simulink model "ImpJoystick"  (R2025b)
settings: Solver=FixedStepAuto  StartTime=0.0  StopTime=inf  FixedStep=Ts  RelTol=1e-3
model workspace (MAT data in the model file):
  SL_ROS_VariableLengthArrays_MaxSizes.CommonInfo.ArrayTruncateAction = 'EmitWarning'
  SL_ROS_VariableLengthArrays_MaxSizes.MsgTypeMap = containers.Map
  SL_ROS_VariableLengthArrays_MaxSizes.MsgTypeMap.serialization.keys = {'sensor_msgs/JointState'}
  SL_ROS_VariableLengthArrays_MaxSizes.MsgTypeMap.serialization.values{1}(1).PropertyName = 'effort'
  SL_ROS_VariableLengthArrays_MaxSizes.MsgTypeMap.serialization.values{1}(1).DataType = 'double'
  SL_ROS_VariableLengthArrays_MaxSizes.MsgTypeMap.serialization.values{1}(1).MaxLength = 3
  SL_ROS_VariableLengthArrays_MaxSizes.MsgTypeMap.serialization.values{1}(2).PropertyName = 'name'
  SL_ROS_VariableLengthArrays_MaxSizes.MsgTypeMap.serialization.values{1}(2).DataType = 'std_msgs/String'
  SL_ROS_VariableLengthArrays_MaxSizes.MsgTypeMap.serialization.values{1}(2).MaxLength = 16
  SL_ROS_VariableLengthArrays_MaxSizes.MsgTypeMap.serialization.values{1}(3).PropertyName = 'position'
  SL_ROS_VariableLengthArrays_MaxSizes.MsgTypeMap.serialization.values{1}(3).DataType = 'double'
  SL_ROS_VariableLengthArrays_MaxSizes.MsgTypeMap.serialization.values{1}(3).MaxLength = 3
  SL_ROS_VariableLengthArrays_MaxSizes.MsgTypeMap.serialization.values{1}(4).PropertyName = 'velocity'
  SL_ROS_VariableLengthArrays_MaxSizes.MsgTypeMap.serialization.values{1}(4).DataType = 'double'
  SL_ROS_VariableLengthArrays_MaxSizes.MsgTypeMap.serialization.values{1}(4).MaxLength = 3
  SL_ROS_VariableLengthArrays_MaxSizes.MsgTypeMap.serialization.uniformity = 0
  SL_ROS_VariableLengthArrays_MaxSizes.MsgTypeMap.serialization.keyType = 'char'
  SL_ROS_VariableLengthArrays_MaxSizes.MsgTypeMap.serialization.valueType = 'any'
values from neighbouring files (symbols this model uses):
  hiddenLayerSizeCtrl = 20    [InitJoystick.m]
  hiddenLayerSizeObsv = 5    [InitJoystick.m]
  p = 3    [InitJoystick.m]
  torque2voltage = voltage_max ./ u_max    [InitJoystick.m]
  Ts = 1e-3    (= 0.001)    [InitJoystick.m]
  u_max = motor_max_torque * gear_ratio    [InitJoystick.m]
  u_min = - motor_max_torque * gear_ratio    [InitJoystick.m]
  Vctrl0 = 0.1 * randn(hiddenLayerSizeCtrl, inputLayerSizeCtrl)    [InitJoystick.m]
  Vobsv0 = 0.1 * randn(hiddenLayerSizeObsv, inputLayerSizeObsv)    [InitJoystick.m]
  Wctrl0 = 0.1 * randn(outputLayerSizeCtrl, hiddenLayerSizeCtrl)    [InitJoystick.m]
  Wobsv0 = 0.1 * randn(outputLayerSizeObsv, hiddenLayerSizeObsv)    [InitJoystick.m]
  x_hat0 = zeros(n, 1)    [InitJoystick.m]
undefined symbols (not defined in the file or in its folder): effort, effort_SL_Info, position, position_SL_Info
libraries: ros2lib x3, slpidlib x3, sl3dlib x1
settings Model: Creator=Asus  LastModifiedBy=Asus
settings OptimizationCC: DefaultParameterBehavior=Inlined  EnhancedBackFolding=on  PassReuseOutputArgsAs=Individual arguments  ZeroExternalMemoryAtStartup=off  ZeroInternalMemoryAtStartup=off  MaxStackSize=64  OptimizeBlockOrder=speed  DifferentSizesBufferReuse=on  OptimizationCustomize=off  EfficientTunableParamExpr=on
settings DebuggingCC: InheritedTsInSrcMsg=none  ParameterTunabilityLossMsg=error
settings SFSimCC: MATLABDynamicMemAlloc=off
settings RTWCC: SystemTargetFile=ert.tlc  HardwareBoard=Robot Operating System 2 (ROS 2)  TLCOptions="-aInlineSetEventsForThisBaseRateFcn=TLC_FALSE -aSuppressMultiTaskScheduler=TLC_FALSE  -aRateBasedStepFcn=0"  TemplateMakefile=ert_default_tmf  Toolchain=Colcon Tools  TargetLang=C++  Description=Embedded Coder
settings CodeAppCC: ForceParamTrailComments=on  IgnoreCustomStorageClasses=off  MaxIdLength=95.0  OperatorAnnotations=on  SimulinkDataObjDesc=on  SFDataObjDesc=on  InsertBlockDesc=on
settings ERTTargetCC: RootIOFormat=Structure reference  CodeInterfacePackaging=C++ class

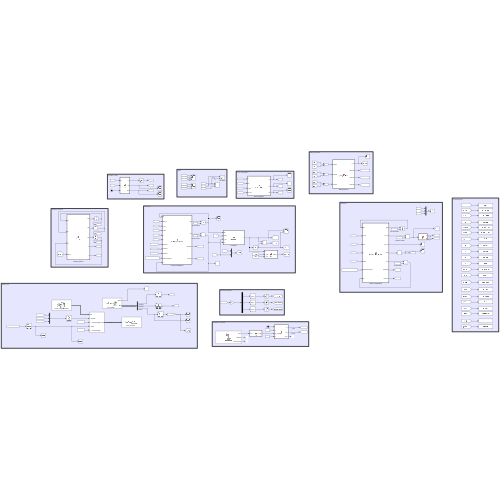
[thumbnail: Simulink's stored preview of the top-level diagram]
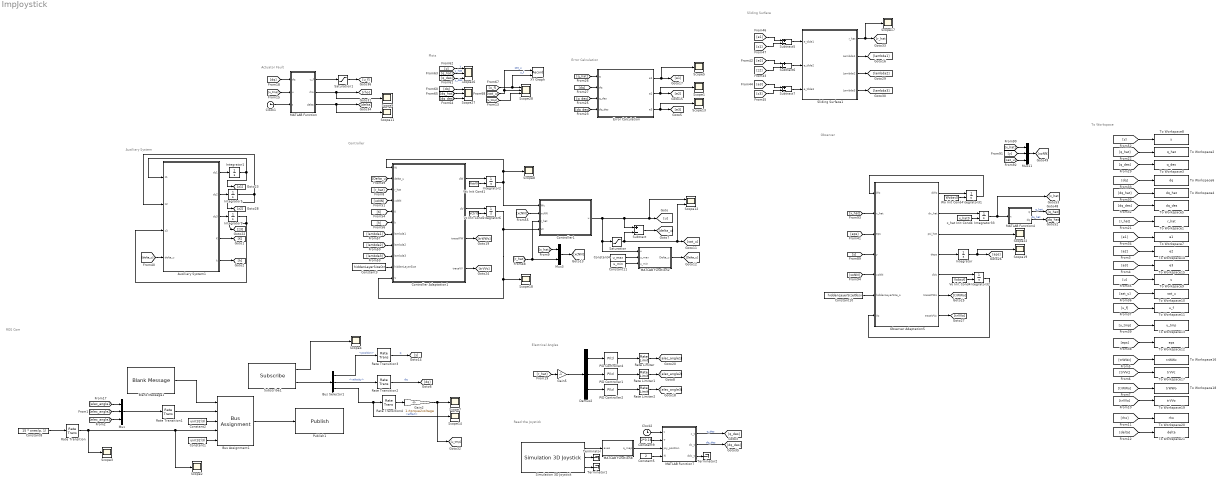
== system ImpJoystick ==
  note: To Workspace
  note: Electrical Angles
  note: Plots
  note: Observer
  note: ROS Com
  note: Actuator Fault
  note: Auxiliary System
  note: Error Calculation
  note: Sliding Surface
  note: Controller
  note: Read the Joystick
  Auxiliary System1 : MATLAB Function  TreatAsAtomicUnit=on
  Blank Message1 : ros2lib/Blank Message  messageClass=Message  entityType=sensor_msgs/JointState  messageType=sensor_msgs/JointState  SampleTime=0.02
  Bus Assignment1 : BusAssignment  AssignedSignals=position,position_SL_Info.CurrentLength,effort,effort_SL_Info.CurrentLength
  Bus Selector1 : BusSelector  OutputSignals=position,velocity,effort
  Clock1 : Clock
  Clock2 : Clock
  Constant1 : Constant  Value=uint32(3)
  Constant10 : Constant  Value=hiddenLayerSizeObsv
  Constant11 : Constant  Value=u_min
  Constant2 : Constant  Value=uint32(3)
  Constant3 : Constant  Value=hiddenLayerSizeCtrl
  Constant4 : Constant  Value=u_max
  Constant5 : Constant  Value=2
  Constant8 : Constant  Value=15 * ones(p, 1)
  Constant9 : Constant  Value=2*0.16
  Controller Adaptation1 : MATLAB Function  TreatAsAtomicUnit=on
  Controller1 : MATLAB Function  TreatAsAtomicUnit=on
  Demux2 : Demux  Outputs=3
  Error Calculation : MATLAB Function  TreatAsAtomicUnit=on
  Gain2 : Gain  Gain=1./torque2voltage
  Gain5 : Gain  Gain=-1
  Integrator : Integrator  InitialCondition=5 * ones(p, 1)
  Integrator1 : Integrator  InitialCondition=zeros(2, 1)
  Integrator{2,6,31..33} (5 alike) : Integrator  InitialConditionSource=external  InitialCondition=[0.5; 0.5]
  Integrator5 : Integrator  InitialCondition=zeros(2, 1)
  Integrator9 : Integrator  InitialCondition=zeros(2, 1)
  MATLAB Function : MATLAB Function  TreatAsAtomicUnit=on
  MATLAB Function2 : MATLAB Function  TreatAsAtomicUnit=on
  MATLAB Function4 : MATLAB Function  TreatAsAtomicUnit=on
  MATLAB Function7 : MATLAB Function  TreatAsAtomicUnit=on  SystemSampleTime=Ts
  MATLAB Function8 : MATLAB Function  TreatAsAtomicUnit=on
  Mux : Mux  Inputs=3
  Mux11 : Mux  Inputs=3
  Mux3 : Mux  Inputs=2
  Observer Adaptation5 : MATLAB Function  TreatAsAtomicUnit=on
  PID Controller1 : slpidlib/PID Controller  Controller=PI  Form=Parallel  TimeDomain=Discrete-time  UseExternalTs=off  SampleTime=-1  IntegratorMethod=Trapezoidal  FilterMethod=Forward Euler  ControllerParametersSource=internal  P=0.05  I=1  UseKiTs=off  D=0  UseExternalDerivativeSource=off  N=100  UseFilter=on  TunerSelectOption=Transfer Function Based (PID Tuner App)  InitialConditionSource=internal  InitialConditionForIntegrator=0  InitialConditionForFilter=0  DifferentiatorICPrevScaledInput=0  ExternalReset=none  TrackingMode=off  Kt=1  LimitOutput=off  SatLimitsSource=internal  UpperSaturationLimit=50  LowerSaturationLimit=-50  LinearizeAsGain=on  AntiWindupMode=none  Kb=1  LimitIntegrator=off  UpperIntegratorSaturationLimit=50  LowerIntegratorSaturationLimit=-50  POutMin=[]  POutMax=[]  IOutMin=[]  IOutMax=[]  DOutMin=[]  DOutMax=[]  NOutMin=[]  NOutMax=[]  SumOutMin=[]  SumOutMax=[]  SaturationOutMin=[]  SaturationOutMax=[]  PParamMin=[]  PParamMax=[]  IParamMin=[]  IParamMax=[]  DParamMin=[]  DParamMax=[]  NParamMin=[]  NParamMax=[]  KbParamMin=[]  KbParamMax=[]  KtParamMin=[]  KtParamMax=[]  KbOutMin=[]  KbOutMax=[]  KtOutMin=[]  KtOutMax=[]  IntegratorOutMin=[]  IntegratorOutMax=[]  FilterOutMin=[]  FilterOutMax=[]  SumI1OutMin=[]  SumI1OutMax=[]  SumI2OutMin=[]  SumI2OutMax=[]  SumI3OutMin=[]  SumI3OutMax=[]  SumI4OutMin=[]  SumI4OutMax=[]  SumDOutMin=[]  SumDOutMax=[]  DifferentiatorOutMin=[]  DifferentiatorOutMax=[]  FilterDiffOutCoefMin=[]  FilterDiffOutCoefMax=[]  ReciprocalOutMin=[]  ReciprocalOutMax=[]  SumDenOutMin=[]  SumDenOutMax=[]  SumNumOutMin=[]  SumNumOutMax=[]  DivideOutMin=[]  DivideOutMax=[]  UdiffTsProdOutMin=[]  UdiffTsProdOutMax=[]  NTsProdOutMin=[]  NTsProdOutMax=[]  UintegralTsProdOutMin=[]  UintegralTsProdOutMax=[]  UngainTsProdOutMin=[]  UngainTsProdOutMax=[]  ClampingZeroOutDataTypeStr=Inherit: Inherit via back propagation  ClampingZeroOutMin=[]  ClampingZeroOutMax=[]  FilterDenConstantOutDataTypeStr=Inherit: Inherit via back propagation  FilterDenConstantOutMin=[]  FilterDenConstantOutMax=[]  PCopyOutDataTypeStr=Inherit: Inherit via back propagation  PCopyOutMin=[]  PCopyOutMax=[]  NCopyOutDataTypeStr=Inherit: Inherit via back propagation  NCopyOutMin=[]  NCopyOutMax=[]  IntegratorContinuousStateAttributes=''  IntegratorStateMustResolveToSignalObject=off  IntegratorRTWStateStorageClass=Auto  FilterContinuousStateAttributes=''  FilterStateMustResolveToSignalObject=off  FilterRTWStateStorageClass=Auto  ParallelPVariant=InternalParameters  IdealPVariant=Disabled  IVariant=InternalParameters  DVariant=Disabled  IntegratorVariant=Discrete  SatVariant=Disabled  AWVariant=Passthrough  PCopyVariant=Disabled  TRVariant=Disabled  FdbkBlocksVariant=Forward  IdealPFdbkVariant=Disabled  SatFdbkVariant=Disabled  DerivativeFilterVariant=Disabled  NVariant=Disabled  NCopyVariant=Disabled_SignalSpec  FilterICVariant=Disabled  IntegratorICVariant=InternalICs  ExternalResetVariant=Disabled  TRSumVariant=Passthrough  SumFdbkVariant=Disabled  SumVariant=Sum_PI  TsampFilterVariant=InternalTs  TsampNgainVariant=Passthrough  TsampIntegralVariant=Disabled_SignalSpec  ExternalSaturationOutDataTypeStr=Inherit: Same as second input  DerivativeSourceVariant=Disabled  PreIntVariant=InternalPreInt
  PID Controller2 : slpidlib/PID Controller  Controller=PI  Form=Parallel  TimeDomain=Discrete-time  UseExternalTs=off  SampleTime=-1  IntegratorMethod=Trapezoidal  FilterMethod=Forward Euler  ControllerParametersSource=internal  P=0.05  I=1  UseKiTs=off  D=0  UseExternalDerivativeSource=off  N=100  UseFilter=on  TunerSelectOption=Transfer Function Based (PID Tuner App)  InitialConditionSource=internal  InitialConditionForIntegrator=0  InitialConditionForFilter=0  DifferentiatorICPrevScaledInput=0  ExternalReset=none  TrackingMode=off  Kt=1  LimitOutput=off  SatLimitsSource=internal  UpperSaturationLimit=50  LowerSaturationLimit=-50  LinearizeAsGain=on  AntiWindupMode=none  Kb=1  LimitIntegrator=off  UpperIntegratorSaturationLimit=50  LowerIntegratorSaturationLimit=-50  POutMin=[]  POutMax=[]  IOutMin=[]  IOutMax=[]  DOutMin=[]  DOutMax=[]  NOutMin=[]  NOutMax=[]  SumOutMin=[]  SumOutMax=[]  SaturationOutMin=[]  SaturationOutMax=[]  PParamMin=[]  PParamMax=[]  IParamMin=[]  IParamMax=[]  DParamMin=[]  DParamMax=[]  NParamMin=[]  NParamMax=[]  KbParamMin=[]  KbParamMax=[]  KtParamMin=[]  KtParamMax=[]  KbOutMin=[]  KbOutMax=[]  KtOutMin=[]  KtOutMax=[]  IntegratorOutMin=[]  IntegratorOutMax=[]  FilterOutMin=[]  FilterOutMax=[]  SumI1OutMin=[]  SumI1OutMax=[]  SumI2OutMin=[]  SumI2OutMax=[]  SumI3OutMin=[]  SumI3OutMax=[]  SumI4OutMin=[]  SumI4OutMax=[]  SumDOutMin=[]  SumDOutMax=[]  DifferentiatorOutMin=[]  DifferentiatorOutMax=[]  FilterDiffOutCoefMin=[]  FilterDiffOutCoefMax=[]  ReciprocalOutMin=[]  ReciprocalOutMax=[]  SumDenOutMin=[]  SumDenOutMax=[]  SumNumOutMin=[]  SumNumOutMax=[]  DivideOutMin=[]  DivideOutMax=[]  UdiffTsProdOutMin=[]  UdiffTsProdOutMax=[]  NTsProdOutMin=[]  NTsProdOutMax=[]  UintegralTsProdOutMin=[]  UintegralTsProdOutMax=[]  UngainTsProdOutMin=[]  UngainTsProdOutMax=[]  ClampingZeroOutDataTypeStr=Inherit: Inherit via back propagation  ClampingZeroOutMin=[]  ClampingZeroOutMax=[]  FilterDenConstantOutDataTypeStr=Inherit: Inherit via back propagation  FilterDenConstantOutMin=[]  FilterDenConstantOutMax=[]  PCopyOutDataTypeStr=Inherit: Inherit via back propagation  PCopyOutMin=[]  PCopyOutMax=[]  NCopyOutDataTypeStr=Inherit: Inherit via back propagation  NCopyOutMin=[]  NCopyOutMax=[]  IntegratorContinuousStateAttributes=''  IntegratorStateMustResolveToSignalObject=off  IntegratorRTWStateStorageClass=Auto  FilterContinuousStateAttributes=''  FilterStateMustResolveToSignalObject=off  FilterRTWStateStorageClass=Auto  ParallelPVariant=InternalParameters  IdealPVariant=Disabled  IVariant=InternalParameters  DVariant=Disabled  IntegratorVariant=Discrete  SatVariant=Disabled  AWVariant=Passthrough  PCopyVariant=Disabled  TRVariant=Disabled  FdbkBlocksVariant=Forward  IdealPFdbkVariant=Disabled  SatFdbkVariant=Disabled  DerivativeFilterVariant=Disabled  NVariant=Disabled  NCopyVariant=Disabled_SignalSpec  FilterICVariant=Disabled  IntegratorICVariant=InternalICs  ExternalResetVariant=Disabled  TRSumVariant=Passthrough  SumFdbkVariant=Disabled  SumVariant=Sum_PI  TsampFilterVariant=InternalTs  TsampNgainVariant=Passthrough  TsampIntegralVariant=Disabled_SignalSpec  ExternalSaturationOutDataTypeStr=Inherit: Same as second input  DerivativeSourceVariant=Disabled  PreIntVariant=InternalPreInt
  PID Controller4 : slpidlib/PID Controller  Controller=PI  Form=Parallel  TimeDomain=Discrete-time  UseExternalTs=off  SampleTime=-1  IntegratorMethod=Trapezoidal  FilterMethod=Forward Euler  ControllerParametersSource=internal  P=0.05  I=1  UseKiTs=off  D=0  UseExternalDerivativeSource=off  N=100  UseFilter=on  TunerSelectOption=Transfer Function Based (PID Tuner App)  InitialConditionSource=internal  InitialConditionForIntegrator=0  InitialConditionForFilter=0  DifferentiatorICPrevScaledInput=0  ExternalReset=none  TrackingMode=off  Kt=1  LimitOutput=off  SatLimitsSource=internal  UpperSaturationLimit=50  LowerSaturationLimit=-50  LinearizeAsGain=on  AntiWindupMode=none  Kb=1  LimitIntegrator=off  UpperIntegratorSaturationLimit=50  LowerIntegratorSaturationLimit=-50  POutMin=[]  POutMax=[]  IOutMin=[]  IOutMax=[]  DOutMin=[]  DOutMax=[]  NOutMin=[]  NOutMax=[]  SumOutMin=[]  SumOutMax=[]  SaturationOutMin=[]  SaturationOutMax=[]  PParamMin=[]  PParamMax=[]  IParamMin=[]  IParamMax=[]  DParamMin=[]  DParamMax=[]  NParamMin=[]  NParamMax=[]  KbParamMin=[]  KbParamMax=[]  KtParamMin=[]  KtParamMax=[]  KbOutMin=[]  KbOutMax=[]  KtOutMin=[]  KtOutMax=[]  IntegratorOutMin=[]  IntegratorOutMax=[]  FilterOutMin=[]  FilterOutMax=[]  SumI1OutMin=[]  SumI1OutMax=[]  SumI2OutMin=[]  SumI2OutMax=[]  SumI3OutMin=[]  SumI3OutMax=[]  SumI4OutMin=[]  SumI4OutMax=[]  SumDOutMin=[]  SumDOutMax=[]  DifferentiatorOutMin=[]  DifferentiatorOutMax=[]  FilterDiffOutCoefMin=[]  FilterDiffOutCoefMax=[]  ReciprocalOutMin=[]  ReciprocalOutMax=[]  SumDenOutMin=[]  SumDenOutMax=[]  SumNumOutMin=[]  SumNumOutMax=[]  DivideOutMin=[]  DivideOutMax=[]  UdiffTsProdOutMin=[]  UdiffTsProdOutMax=[]  NTsProdOutMin=[]  NTsProdOutMax=[]  UintegralTsProdOutMin=[]  UintegralTsProdOutMax=[]  UngainTsProdOutMin=[]  UngainTsProdOutMax=[]  ClampingZeroOutDataTypeStr=Inherit: Inherit via back propagation  ClampingZeroOutMin=[]  ClampingZeroOutMax=[]  FilterDenConstantOutDataTypeStr=Inherit: Inherit via back propagation  FilterDenConstantOutMin=[]  FilterDenConstantOutMax=[]  PCopyOutDataTypeStr=Inherit: Inherit via back propagation  PCopyOutMin=[]  PCopyOutMax=[]  NCopyOutDataTypeStr=Inherit: Inherit via back propagation  NCopyOutMin=[]  NCopyOutMax=[]  IntegratorContinuousStateAttributes=''  IntegratorStateMustResolveToSignalObject=off  IntegratorRTWStateStorageClass=Auto  FilterContinuousStateAttributes=''  FilterStateMustResolveToSignalObject=off  FilterRTWStateStorageClass=Auto  ParallelPVariant=InternalParameters  IdealPVariant=Disabled  IVariant=InternalParameters  DVariant=Disabled  IntegratorVariant=Discrete  SatVariant=Disabled  AWVariant=Passthrough  PCopyVariant=Disabled  TRVariant=Disabled  FdbkBlocksVariant=Forward  IdealPFdbkVariant=Disabled  SatFdbkVariant=Disabled  DerivativeFilterVariant=Disabled  NVariant=Disabled  NCopyVariant=Disabled_SignalSpec  FilterICVariant=Disabled  IntegratorICVariant=InternalICs  ExternalResetVariant=Disabled  TRSumVariant=Passthrough  SumFdbkVariant=Disabled  SumVariant=Sum_PI  TsampFilterVariant=InternalTs  TsampNgainVariant=Passthrough  TsampIntegralVariant=Disabled_SignalSpec  ExternalSaturationOutDataTypeStr=Inherit: Same as second input  DerivativeSourceVariant=Disabled  PreIntVariant=InternalPreInt
  Publish1 : ros2lib/Publish  topicSource=Specify your own  topic=/joint_desireds  messageType=sensor_msgs/JointState  QOSHistory=Keep last  QOSDepth=10  QOSReliability=Reliable  QOSDurability=Volatile  QOSDeadline=Inf  QOSLifespan=Inf  QOSLiveliness=Automatic  QOSLeaseDuration=Inf  QOSAvoidROSNamespaceConventions=off
  Rate Limiter : RateLimiter  RisingSlewLimit=50  FallingSlewLimit=-50
  Rate Limiter1 : RateLimiter  RisingSlewLimit=50  FallingSlewLimit=-50  SampleTimeMode=inherited
  Rate Limiter2 : RateLimiter  RisingSlewLimit=50  FallingSlewLimit=-50  SampleTimeMode=inherited
  Rate Transition : RateTransition  OutPortSampleTime=0.02
  Rate Transition1 : RateTransition  OutPortSampleTime=0.02
  Rate Transition2 : RateTransition  OutPortSampleTime=Ts
  Rate Transition3 : RateTransition  OutPortSampleTime=Ts
  Rate Transition4 : RateTransition  OutPortSampleTime=Ts
  Saturation : Saturate  UpperLimit=u_max  LowerLimit=u_min
  Saturation1 : Saturate  UpperLimit=u_max  LowerLimit=u_min
  Scope{1..5,7..9,11,13..14,17..19,22} (15 alike) : Scope
      Scope1 settings: ActiveDisplayYMinimum=-0.24287807344006263  ActiveDisplayYMaximum=0.25287974310957717  DataLoggingVariableName=ScopeData3
      Scope11 settings: ActiveDisplayYMinimum=-1  ActiveDisplayYMaximum=1  DataLoggingVariableName=ScopeData6
      Scope13 settings: ActiveDisplayYMinimum=-0.29897924911149121  ActiveDisplayYMaximum=0.2090765790905024  DataLoggingVariableName=ScopeData13
      Scope14 settings: ActiveDisplayYMinimum=-12.649985074996948  ActiveDisplayYMaximum=12.652279615402222  DataLoggingVariableName=ScopeData14
      Scope17 settings: ActiveDisplayYMinimum=-6.84986892680592  ActiveDisplayYMaximum=3.4555315948976819  DataLoggingVariableName=ScopeData19
      Scope18 settings: ActiveDisplayYMinimum=-1  ActiveDisplayYMaximum=1  DataLoggingVariableName=ScopeData10
      Scope19 settings: ActiveDisplayYMinimum=-0.056716812017258533  ActiveDisplayYMaximum=20.510451308155332  DataLoggingVariableName=ScopeData15
      Scope2 settings: ActiveDisplayYMinimum=-1.8749999999999996  ActiveDisplayYMaximum=16.875
      Scope22 settings: ActiveDisplayYMinimum=-0.42606678523590263  ActiveDisplayYMaximum=0.48150686097965856  DataLoggingVariableName=ScopeData18
      Scope3 settings: ActiveDisplayYMinimum=5  ActiveDisplayYMaximum=25  DataLoggingVariableName=ScopeData4
      Scope4 settings: ActiveDisplayYMinimum=-0.12499999999999997  ActiveDisplayYMaximum=1.125  DataLoggingVariableName=ScopeData11
      Scope5 settings: ActiveDisplayYMinimum=-5.0160610234879295  ActiveDisplayYMaximum=4.3832959736672761
      Scope7 settings: ActiveDisplayYMinimum=-4.6454817136128748  ActiveDisplayYMaximum=4.6375481605529787  DataLoggingVariableName=ScopeData8
      Scope8 settings: ActiveDisplayYMinimum=-68.998192796896234  ActiveDisplayYMaximum=67.9276309158068  DataLoggingVariableName=ScopeData20
      Scope9 settings: ActiveDisplayYMinimum=0.89735957983734793  ActiveDisplayYMaximum=1.3932448974534157  DataLoggingVariableName=ScopeData5
  Scope12 : Scope  NumInputPorts=2
      settings: ActiveDisplayYMinimum=-6.9909348188181673  ActiveDisplayYMaximum=6.9347067315860729  DataLoggingVariableName=ScopeData7
  Scope26 : Scope  NumInputPorts=3
      settings: ActiveDisplayYMinimum=-0.16267971265796272  ActiveDisplayYMaximum=0.24936946493277015  DataLoggingVariableName=ScopeData22
  Scope27 : Scope  NumInputPorts=3
      settings: ActiveDisplayYMinimum=-0.15237484375  ActiveDisplayYMaximum=0.27574859375000021  DataLoggingVariableName=ScopeData23
  Scope28 : Scope  NumInputPorts=3
      settings: ActiveDisplayYMinimum=-1.7792114485048884  ActiveDisplayYMaximum=0.75655926497715087  DataLoggingVariableName=ScopeData24
  Simulation 3D Joystick : sl3dlib/Simulation 3D/Hardware Interface/Simulation 3D Joystick  joyid=1  adjustports=on  forcefeed=off
  Sliding Surface1 : MATLAB Function  TreatAsAtomicUnit=on
  Subscribe1 : ros2lib/Subscribe  topicSource=Select from ROS network  topic=/joint_states  messageType=sensor_msgs/JointState  sampleTime=0.02  QOSHistory=Keep all  QOSDepth=3  QOSReliability=Best effort  QOSDurability=Volatile  QOSDeadline=Inf  QOSLifespan=Inf  QOSLiveliness=Automatic  QOSLeaseDuration=Inf  QOSAvoidROSNamespaceConventions=off
  Subtract{,5..7} (4 alike) : Sum  Inputs=+-
  Terminator : Terminator
  Terminator1 : Terminator
  Terminator2 : Terminator
  To Workspace1 : ToWorkspace  VariableName=r_hat  SaveFormat=Structure  SampleTime=-1
      settings: Save2DSignal=2-D array (concatenate along first dimension)
  To Workspace10 : ToWorkspace  VariableName=sat_u  SaveFormat=Structure  SampleTime=-1
      settings: Save2DSignal=2-D array (concatenate along first dimension)
  To Workspace11 : ToWorkspace  VariableName=u_f  SaveFormat=Structure  SampleTime=-1
      settings: Save2DSignal=2-D array (concatenate along first dimension)
  To Workspace12 : ToWorkspace  VariableName=eps  SaveFormat=Structure  SampleTime=-1
      settings: Save2DSignal=2-D array (concatenate along first dimension)
  To Workspace13 : ToWorkspace  VariableName=u_tmp  SaveFormat=Structure  SampleTime=-1
      settings: Save2DSignal=2-D array (concatenate along first dimension)
  To Workspace14 : ToWorkspace  VariableName=e2  SaveFormat=Structure  SampleTime=-1
      settings: Save2DSignal=2-D array (concatenate along first dimension)
  To Workspace15 : ToWorkspace  VariableName=e3  SaveFormat=Structure  SampleTime=-1
      settings: Save2DSignal=2-D array (concatenate along first dimension)
  To Workspace16 : ToWorkspace  VariableName=trWWc  SaveFormat=Structure  SampleTime=-1
      settings: Save2DSignal=2-D array (concatenate along first dimension)
  To Workspace17 : ToWorkspace  VariableName=trVVc  SaveFormat=Structure  SampleTime=-1
      settings: Save2DSignal=2-D array (concatenate along first dimension)
  To Workspace18 : ToWorkspace  VariableName=trWWo  SaveFormat=Structure  SampleTime=-1
      settings: Save2DSignal=2-D array (concatenate along first dimension)
  To Workspace19 : ToWorkspace  VariableName=trVVo  SaveFormat=Structure  SampleTime=-1
      settings: Save2DSignal=2-D array (concatenate along first dimension)
  To Workspace2 : ToWorkspace  VariableName=q_hat  SaveFormat=Structure  SampleTime=-1
      settings: Save2DSignal=2-D array (concatenate along first dimension)
  To Workspace20 : ToWorkspace  VariableName=rho  SaveFormat=Structure  SampleTime=-1
      settings: Save2DSignal=2-D array (concatenate along first dimension)
  To Workspace21 : ToWorkspace  VariableName=delta  SaveFormat=Structure  SampleTime=-1
      settings: Save2DSignal=2-D array (concatenate along first dimension)
  To Workspace3 : ToWorkspace  VariableName=q_des  SaveFormat=Structure  SampleTime=-1
      settings: Save2DSignal=2-D array (concatenate along first dimension)
  To Workspace4 : ToWorkspace  VariableName=dq_hat  SaveFormat=Structure  SampleTime=-1
      settings: Save2DSignal=2-D array (concatenate along first dimension)
  To Workspace5 : ToWorkspace  VariableName=dq_des  SaveFormat=Structure  SampleTime=-1
      settings: Save2DSignal=2-D array (concatenate along first dimension)
  To Workspace6 : ToWorkspace  VariableName=dq  SaveFormat=Structure  SampleTime=-1
      settings: Save2DSignal=2-D array (concatenate along first dimension)
  To Workspace7 : ToWorkspace  VariableName=e1  SaveFormat=Structure  SampleTime=-1
      settings: Save2DSignal=2-D array (concatenate along first dimension)
  To Workspace8 : ToWorkspace  VariableName=y  SaveFormat=Structure  SampleTime=-1
      settings: Save2DSignal=2-D array (concatenate along first dimension)
  To Workspace9 : ToWorkspace  VariableName=u  SaveFormat=Structure  SampleTime=-1
      settings: Save2DSignal=2-D array (concatenate along first dimension)
  Vc Init Cond1 : Constant  Value=Vctrl0
  Vo Init Cond4 : Constant  Value=Vobsv0
  Wc Init Cond1 : Constant  Value=Wctrl0
  Wo Init Cond4 : Constant  Value=Wobsv0
  XY Graph : Record  NumPorts=2.0  FileSettingsInternal="{\"entries\":[{\"content\":{\"excelSettings\":{\"content\":{},\"type\":\"Streamout.ExcelSettings\"},\"parquetSettings\":{\"content\":{},\"type\":\"Streamout.ParquetSettings\"}},\"type\":\"Streamout.FileSettingStorage\",\"uuid\":\"\"}],\"packageUris\":[\"http:\\/\\/schema.mathworks.com\\/mf0\\/streamout_blocks\\/R2020a\"],\"version\":\"1.0\"}"  FrameSettings=[0, 0]  Layout=[1 1]  SignalsInternal="{\"entries\":[{\"content\":{\"signals\":[{\"content\":{\"blockPath\":[],\"dimensions\":[3,1],\"domain\":\"\",\"hasChildren\":true,\"lineColor\":\"#ff6929\",\"lineWidth\":2,\"port\":1,\"signalID\":1,\"signalName\":\"sat_u\"},\"type\":\"RecordBlkView.Signal\",\"uuid\":\"\"},{\"content\":{\"blockPath\":[],\"channel\":[1,1],\"dimensions\":[3,1],\"domain\":\"\",\"lineColor\":\"#64d413\",\"lineWidth\":2,\"parentID\":1,\"port\":1,\"signalID\":2,\"signalName\":\"sat_u\"},\"type\":\"RecordBlkView.Signal\",\"uuid\":\"\"},{\"content\":{\"blockPath\":[],\"channel\":[2,1],\"dimensions\":[3,1],\"domain\":\"\",\"lineColor\":\"#d95319\",\"lineWidth\":2,\"parentID\":1,\"plots\":[ 1 ],\"port\":1,\"signalID\":3,\"signalName\":\"sat_u\"},\"type\":\"RecordBlkView.Signal\",\"uuid\":\"\"},{\"content\":{\"blockPath\":[],\"channel\":[3,1],\"dimensions\":[3,1],\"domain\":\"\",\"lineColor\":\"#edb120\",\"lineWidth\":2,\"parentID\":1,\"port\":1,\"signalID\":4,\"signalName\":\"sat_u\"},\"type\":\"RecordBlkView.Signal\",\"uuid\":\"\"},{\"content\":{\"blockPath\":[],\"dimensions\":[3,1],\"domain\":\"\",\"hasChildren\":true,\"lineColor\":\"#64d413\",\"lineWidth\":2,\"port\":2,\"signalID\":5,\"signalName\":\"u_f\"},\"type\":\"RecordBlkView.Signal\",\"uuid\":\"\"},{\"content\":{\"blockPath\":[],\"channel\":[1,1],\"dimensions\":[3,1],\"domain\":\"\",\"lineColor\":\"#fe330a\",\"lineWidth\":2,\"parentID\":5,\"port\":2,\"signalID\":6,\"signalName\":\"u_f\"},\"type\":\"RecordBlkView.Signal\",\"uuid\":\"\"},{\"content\":{\"blockPath\":[],\"channel\":[2,1],\"dimensions\":[3,1],\"domain\":\"\",\"lineColor\":\"#7e2f8e\",\"lineWidth\":2,\"parentID\":5,\"plots\":[ 1 ],\"port\":2,\"signalID\":7,\"signalName\":\"u_f\"},\"type\":\"RecordBlkView.Signal\",\"uuid\":\"\"},{\"content\":{\"blockPath\":[],\"channel\":[3,1],\"dimensions\":[3,1],\"domain\":\"\",\"lineColor\":\"#77ac30\",\"lineWidth\":2,\"parentID\":5,\"port\":2,\"signalID\":8,\"signalName\":\"u_f\"},\"type\":\"RecordBlkView.Signal\",\"uuid\":\"\"}]},\"type\":\"RecordBlkView.InputSignals\",\"uuid\":\"\"}],\"packageUris\":[\"http:\\/\\/schema.mathworks.com\\/mf0\\/streamout_blocks\\/R2020a\"],\"version\":\"1.0\"}"  VisualizationBindings="{\"xyplotplugin\":{\"info\":[{\"series\":[{\"bindingParametersList\":[{\"parameter\":\"X-Axis\",\"signalID\":3,\"signalName\":\"sat_u(2,1)\"},{\"parameter\":\"Y-Axis\",\"signalID\":7,\"signalName\":\"u_f(2,1)\"}],\"seriesID\":0}],\"subplotID\":1}]}}"  CompatibilityTag=XY
  x_hat Init Cond4 : Constant  Value=x_hat0
  wires:
  Mux/1 -> Rate Transition1/1
  Blank Message1/1 -> Bus Assignment1/1
  Integrator31/1 -> Observer Adaptation5/1(Wo)
  Wo Init Cond4/1 -> Integrator31/2
  Bus Selector1/2 -> Rate Transition2/1  "<velocity>"
  Observer Adaptation5/4(deps) -> Integrator/1
  Vo Init Cond4/1 -> Integrator32/2
  [x_hat] -> Observer Adaptation5/2(x_hat)
  [dq] -> MATLAB Function/1(dq)
  Bus Assignment1/1 -> Publish1/1
  MATLAB Function/2(rho) -> [rho], Scope9/1
  [y] -> Observer Adaptation5/4(y)
  MATLAB Function/3(delta) -> [delta], Scope11/1
  [eps] -> Observer Adaptation5/3(eps)
  [sat_u] -> Mux11/3
  Clock1/1 -> MATLAB Function/3(t)
  [dq_des] -> Scope27/3
  MATLAB Function4/1(q) -> [q_hat]  "q_hat"
  [u_tmp] -> MATLAB Function/2(u)
  Bus Selector1/1 -> Rate Transition3/1  "<position>"
  [q_des] -> Scope26/3  "y_des"
  Rate Transition1/1 -> Bus Assignment1/2
  Observer Adaptation5/1(dWo) -> Integrator31/1
  Constant1/1 -> Bus Assignment1/5
  MATLAB Function/1(u_f) -> Saturation1/1
  Constant10/1 -> Observer Adaptation5/6(hiddenLayerSize_o)
  [x_hat] -> Mux11/1
  [y] -> Mux11/2
  Integrator/1 -> Scope19/1, [eps]
  Observer Adaptation5/2(dx_hat) -> Integrator33/1
  Integrator32/1 -> Observer Adaptation5/7(Vo)
  MATLAB Function4/2(dq) -> [dq_hat]  "dq_hat"
  Subscribe1/1 -> Scope4/1
  [dq] -> Scope27/1
  [q_hat] -> Scope26/2  "y_hat"
  [u_f] -> XY Graph/2, Scope28/1  "u_f"
  [dq_hat] -> Scope27/2
  Subscribe1/2 -> Bus Selector1/1
  [xoNN] -> Observer Adaptation5/5(xoNN)
  x_hat Init Cond4/1 -> Integrator33/2
  [y] -> Scope26/1  "y"
  Observer Adaptation5/3(psi_hat) -> Scope22/1
  Saturation1/1 -> [u_f]
  [sat_u] -> XY Graph/1, Scope28/2  "sat_u"
  Mux11/1 -> [xoNN]
  Rate Transition4/1 -> Gain2/1
  Observer Adaptation5/5(dVo) -> Integrator32/1
  Bus Selector1/3 -> Scope14/1, Rate Transition4/1  "<effort>"
  Constant2/1 -> Bus Assignment1/3
  Integrator33/1 -> MATLAB Function4/1(x), [x_hat]
  Gain2/1 -> [u_tmp], Scope7/1
  Rate Transition/1 -> Scope2/1, Bus Assignment1/4, Scope3/1
  Rate Limiter/1 -> [elec_angle1]
  PID Controller4/1 -> Rate Limiter/1
  [y] -> To Workspace8/1
  [r_hat] -> To Workspace1/1
  [q_hat] -> To Workspace2/1
  [q_des] -> To Workspace3/1
  [dq_hat] -> To Workspace4/1
  [dq] -> To Workspace6/1
  [dq_des] -> To Workspace5/1
  [e1] -> To Workspace7/1
  [u] -> To Workspace9/1
  [sat_u] -> To Workspace10/1
  [u_f] -> To Workspace11/1
  [eps] -> To Workspace12/1
  [u_tmp] -> To Workspace13/1
  Auxiliary System1/1(dz1) -> Integrator1/1
  Auxiliary System1/3(dz3) -> Integrator9/1
  Auxiliary System1/2(dz2) -> Integrator5/1
  Integrator5/1 -> [z2], Auxiliary System1/2(z2)
  Auxiliary System1/5(h) -> [h]
  Integrator9/1 -> Auxiliary System1/3(z3), [z3]
  [delta_u] -> Auxiliary System1/4(delta_u)
  Integrator1/1 -> [z1], Auxiliary System1/1(z1)
  Auxiliary System1/4(K) -> [K]
  Error Calculation/2(e2) -> [e2], Scope1/1
  Error Calculation/1(e1) -> [e1], Scope5/1
  Error Calculation/3(e3) -> Scope13/1, [e3]
  [dq] -> Error Calculation/2(dq)
  [dq_des] -> Error Calculation/4(dq_des)
  [q_hat] -> Error Calculation/1(q)
  [q_des] -> Error Calculation/3(q_des)
  [z1] -> Subtract5/2
  Subtract6/1 -> Sliding Surface1/2(e_tilde2)
  [z3] -> Subtract7/2
  Sliding Surface1/3(Lambda2) -> [lambda2]
  Sliding Surface1/4(Lambda3) -> [lambda3]
  Sliding Surface1/2(Lambda1) -> [lambda1]
  Subtract7/1 -> Sliding Surface1/3(e_tilde3)
  Subtract5/1 -> Sliding Surface1/1(e_tilde1)
  Sliding Surface1/1(r_hat) -> Scope17/1, [r_hat]
  [e3] -> Subtract7/1
  [e1] -> Subtract5/1
  [e2] -> Subtract6/1
  [z2] -> Subtract6/2
  [r_hat] -> Controller Adaptation1/3(r_hat)
  Controller Adaptation1/2(dV) -> Integrator6/1
  MATLAB Function2/1(Delta_u) -> [Delta_u]
  Integrator2/1 -> Controller1/1(Wc), Scope8/1, Controller Adaptation1/1(W)
  [lambda3] -> Controller Adaptation1/9(lambda3)
  [xcNN] -> Controller Adaptation1/4(xcNN)
  Controller Adaptation1/1(dW) -> Integrator2/1
  Constant4/1 -> MATLAB Function2/2(u_max)
  [lambda2] -> Controller Adaptation1/8(lambda2)
  [r_hat] -> Controller1/3(r_hat), Mux3/2
  [Delta_u] -> Controller Adaptation1/2(delta_u)
  Constant11/1 -> MATLAB Function2/3(u_min)
  [lambda1] -> Controller Adaptation1/7(lambda1)
  Wc Init Cond1/1 -> Integrator2/2
  Subtract/1 -> [delta_u]
  [h] -> Controller Adaptation1/6(h)
  Vc Init Cond1/1 -> Integrator6/2
  Mux3/1 -> [xcNN]
  [xcNN] -> Controller1/2(xcNN)
  Controller1/1(u) -> Scope12/1, [u], Subtract/1, MATLAB Function2/1(u), Saturation/1
  [x_hat] -> Mux3/1
  [K] -> Controller Adaptation1/5(K)
  Constant3/1 -> Controller Adaptation1/10(hiddenLayerSize)
  Integrator6/1 -> Scope18/1, Controller Adaptation1/11(V), Controller1/4(Vc)
  Saturation/1 -> Scope12/2, [sat_u], Subtract/2
  PID Controller1/1 -> Rate Limiter1/1
  Rate Limiter1/1 -> [elec_angle2]
  PID Controller2/1 -> Rate Limiter2/1
  Rate Limiter2/1 -> [elec_angle3]
  [elec_angle3] -> Mux/3
  [elec_angle2] -> Mux/2
  [e2] -> To Workspace14/1
  [e3] -> To Workspace15/1
  Rate Transition3/1 -> [y]  "q"
  Rate Transition2/1 -> [dq]  "dq"
  Controller Adaptation1/3(traceWW) -> [trWWc]
  Controller Adaptation1/4(traceVV) -> [trVVc]
  Observer Adaptation5/6(traceWWo) -> [trWWo]
  Observer Adaptation5/7(traceVVo) -> [trVVo]
  [trWWc] -> To Workspace16/1
  [trVVc] -> To Workspace17/1
  [trVVo] -> To Workspace19/1
  [trWWo] -> To Workspace18/1
  [rho] -> To Workspace20/1
  [delta] -> To Workspace21/1
  [elec_angle1] -> Mux/1
  Constant8/1 -> Rate Transition/1
  Demux2/1 -> PID Controller4/1
  Demux2/2 -> PID Controller1/1
  Demux2/3 -> PID Controller2/1
  Simulation 3D Joystick/1 -> MATLAB Function8/1(axes)
  Constant9/1 -> MATLAB Function7/2(T)
  MATLAB Function7/3(ddx_t) -> Terminator2/1
  Simulation 3D Joystick/3 -> Terminator1/1
  Simulation 3D Joystick/2 -> Terminator/1
  MATLAB Function8/1(q_map) -> MATLAB Function7/3(joy_position)
  Clock2/1 -> MATLAB Function7/1(t)
  [u_tmp] -> Scope28/3
  MATLAB Function7/1(x_t) -> [q_des]  "q_des"
  Constant5/1 -> MATLAB Function7/4(N)
  MATLAB Function7/2(dx_t) -> [dq_des]  "dq_des"
  [r_hat] -> Gain5/1
  Gain5/1 -> Demux2/1

== matlab function ImpJoystick/Controller Adaptation1 ==
  data: dW output; dV output; W input; delta_u input; r_hat input; xcNN input; K input; h input; lambda1 input; lambda2 input; lambda3 input; hiddenLayerSize input; V input; traceWW output; traceVV output
function [dW, dV, traceWW, traceVV] = ControllerAdaptation(W, delta_u, r_hat, xcNN, K, h, lambda1, lambda2, lambda3, hiddenLayerSize, V)
    
    Sigma = @(z) (-1 + 2 ./ (1 + exp(-2 * z)));


    l = 20 * [2; 2; 2];

    A1 = [0, 1; 0, 0];
    A2 = [0, 1; 0, 0];
    A3 = [0, 1; 0, 0];

    B1 = [0; 1];
    B2 = [0; 1];
    B3 = [0; 1];

    Ac1 = A1 - B1 * ([lambda1', 1] * l(1) + [0, lambda1']);
    Ac2 = A2 - B2 * ([lambda2', 1] * l(2) + [0, lambda2']);
    Ac3 = A3 - B3 * ([lambda3', 1] * l(3) + [0, lambda3']);

    Ac = blkdiag(Ac1, Ac2, Ac3);
    B  = blkdiag(B1, B2, B3);

    eta   = 10 * [0.1, 0.1];
    gamma = [0.0001, 0.0001];

    PI_c      = diag(Sigma(V * xcNN).^2);
    PI_lambda = blkdiag([lambda1', 1], [lambda2', 1], [lambda3', 1]);
    
    dW = eta(1) * (r_hat' * PI_lambda * (-Ac^(-1) * B + K^(-1) * h * diag(delta_u)))' * Sigma(V * xcNN)' - gamma(1) * norm(r_hat) * W;
    dV = eta(2) * (r_hat' * PI_lambda * (-Ac^(-1) * B + K^(-1) * h * diag(delta_u)) * W * (eye(20) - PI_c))' * xcNN' - gamma(2) * norm(r_hat) * V;

    traceWW = trace(W' * W);
    traceVV = trace(V' * V);

end

== matlab function ImpJoystick/Error Calculation ==
  data: e1 output; e2 output; q input; dq input; q_des input; dq_des input; e3 output
function [e1, e2, e3] = ErrorCalculation(q, dq, q_des, dq_des)

    % e1 = zeros(2, 1);
    % e2 = zeros(2, 1);
    % e3 = zeros(2, 1);

    y_bar1 = [q(1); dq(1)];
    y_bar2 = [q(2); dq(2)];
    y_bar3 = [q(3); dq(3)];

    y_bar_des1 = [q_des(1); dq_des(1)];
    y_bar_des2 = [q_des(2); dq_des(2)];
    y_bar_des3 = [q_des(3); dq_des(3)];

    e1 = y_bar1 - y_bar_des1;
    e2 = y_bar2 - y_bar_des2;
    e3 = y_bar3 - y_bar_des3;
    
end

== matlab function ImpJoystick/Auxiliary System1 ==
  data: z1 input; z2 input; z3 input; dz1 output; delta_u input; dz2 output; dz3 output; K output; h output
function [dz1, dz2, dz3, K, h] = AuxiliarySystem(z1, z2, z3, delta_u)
    
    K1  = 1000 * diag([-1, -2]); K2  = 1000 * diag([-1, -2]); K3  = 1000 * diag([-1, -2]);
    h1  = - 5 * [-1; -1]; h2  = - 5 * [-1; -1]; h3  = - 5 * [-1; -1];
    
    K = blkdiag(K1, K2, K3);
    h = blkdiag(h1, h2, h3);

    dz1 = K1 * z1 + h1 * delta_u(1);
    dz2 = K2 * z2 + h2 * delta_u(2);
    dz3 = K3 * z3 + h3 * delta_u(3);
    
end

== matlab function ImpJoystick/MATLAB Function8 ==
  data: axes input; q_map output
function q_map = fcn(axes)

    scales = [-0.25, 0.5, 1.0];
    q_map  = fliplr(axes(1:3)' .* scales)';

end

== matlab function ImpJoystick/Controller1 ==
  data: u output; Wc input; xcNN input; r_hat input; Vc input
function u = Controller(Wc, xcNN, r_hat, Vc)

    Sigma = @(z) (-1 + 2 ./ (1 + exp(-2 * z)));

    K   = 0 * diag([1, 1, 1]);

    u = - Wc * Sigma(Vc * xcNN) - K * r_hat;
    
end

== matlab function ImpJoystick/MATLAB Function2 ==
  data: u input; Delta_u output; u_max input; u_min input
function Delta_u = fcn(u, u_max, u_min)

    Delta_u = zeros(3, 1);
    for i = 1:3
        if u(i) > u_max(i)
            Delta_u(i)   = 1;
        elseif u(i) < u_min(i)
            Delta_u(i)   = 1;
        else
            Delta_u(i)   = 0;
        end
    end

end

== matlab function ImpJoystick/MATLAB Function4 ==
  data: x input; q output; dq output
function [q, dq] = fcn(x)

    q  = x([1, 3, 5]);
    dq = x([2, 4, 6]);

end

== matlab function ImpJoystick/Observer Adaptation5 ==
  data: dWo output; dx_hat output; psi_hat output; deps output; dVo output; Wo input; x_hat input; eps input; y input; xoNN input; hiddenLayerSize_o input; Vo input; traceWWo output; traceVVo output
function [dWo, dx_hat, psi_hat, deps, dVo, traceWWo, traceVVo] = ObserverAdaptation(Wo, x_hat, eps, y, xoNN, hiddenLayerSize_o, Vo)

    Sigma = @(z) (-1 + 2 ./ (1 + exp(-2 * z)));
    Sigma_o = Sigma(Vo * xoNN);


    B1    = [0; 1]; B2 = [0; 1]; B3 = [0; 1];
    C1    = [1; 0]; C2 = [1; 0]; C3 = [1; 0];

    B     = blkdiag(B1, B2, B3);
    C     = blkdiag(C1, C2, C3);
    
    A1 = [0, 1; 0, 0];
    A2 = [0, 1; 0, 0];
    A3 = [0, 1; 0, 0];
    A  = blkdiag(A1, A2, A3);

    y_hat   = C' * x_hat;
    y_tilde = y - y_hat;

    alpha  = [2, 10; 2, 10; 2, 10];
    lambda = [0.01; 0.01; 0.01];
    kappa  = 100 ./ lambda;
    deps   = zeros(3, 1);
    for i  = 1:3
        if abs(y_tilde(i)) > lambda(i)
            deps(i) = kappa(i) * y_tilde(i)^2;
        end
    end
    
    rho1 = 2; rho2 = 2; rho3 = 2;
    Ho = diag([alpha(1, 2)*eps(1)^rho1; alpha(2, 2)*eps(2)^rho2; alpha(3, 2)*eps(3)^rho3]);
    
    D1 = [alpha(1, 1)*eps(1); 0]; D2 = [alpha(2, 1)*eps(2); 0]; D3 = [alpha(3, 1)*eps(3); 0];
    D  = blkdiag(D1, D2, D3);

    Ao   = A  - D*C';
    Aocl = Ao - B*Ho*C';

    psi_hat = Wo * Sigma_o;
    dx_hat  = Ao * x_hat + B * (psi_hat + Ho * y_tilde) + D * y;

    eta_o   = 5 * [10, 10];
    gamma_o = 1 * [0.01, 0.01];

    PI_o = diag(Sigma_o.^2);

    dWo = - eta_o(1) * (y_tilde' * C' * Aocl^(-1) * B)' * Sigma_o' - gamma_o(1) * norm(y_tilde) * Wo;
    dVo = - eta_o(2) * (y_tilde' * C' * Aocl^(-1) * B * Wo * (eye(5) - PI_o))' * xoNN' - gamma_o(2) * norm(y_tilde) * Vo;

    traceWWo = trace(Wo' * Wo);
    traceVVo = trace(Vo' * Vo);

end

== matlab function ImpJoystick/Sliding Surface1 ==
  data: e_tilde1 input; r_hat output; e_tilde2 input; Lambda1 output; e_tilde3 input; Lambda2 output; Lambda3 output
function [r_hat, Lambda1, Lambda2, Lambda3] = SlidingSurface(e_tilde1, e_tilde2, e_tilde3)

    Lambda1 = 50; Lambda2 = 50; Lambda3 = 50;

    r_hat1  = [Lambda1, 1] * e_tilde1;
    r_hat2  = [Lambda2, 1] * e_tilde2;
    r_hat3  = [Lambda3, 1] * e_tilde3;

    r_hat   = [r_hat1; r_hat2; r_hat3];
    
end

== matlab function ImpJoystick/MATLAB Function ==
  data: dq input; u input; u_f output; t input; rho output; delta output
function [u_f, rho, delta] = fcn(dq, u, t)

    t01    = 10;
    rho1   = 0.73 + 0.27 * exp(-0.05 * (t-t01)) - 0.13 * tanh(abs(dq(1)) / 1.5);
    delta1 = -0.45 * tanh(dq(1)) - 0.17 * dq(1);

    t02    = 15;
    rho2   = 0.75 + 0.25 * exp(-0.05 * (t-t02)) - 0.08 * tanh(abs(dq(2)) / 2.5);
    delta2 = 0.64 * tanh(dq(2)) - 0.21 * dq(2);

    t03    = 20;
    rho3   = 0.80 + 0.20 * exp(-0.05 * (t-t03)) + 0.15 * tanh(abs(dq(3)) / 0.95);
    delta3 = - 0.71 * tanh(dq(3)) - 0.32 * dq(3);

    u_f = zeros(3, 1);

    if t < t01
        u_f(1) = u(1);
    else
        u_f(1) = rho1 * u(1) + delta1;
    end

    if t < t02
        u_f(2) = u(2);
    else
        u_f(2) = rho2 * u(2) + delta2;
    end

    if t < t03
        u_f(3) = u(3);
    else
        u_f(3) = rho3 * u(3) + delta3;
    end

    rho   = [rho1; rho2; rho3];
    delta = [delta1; delta2; delta3];


end

== matlab function ImpJoystick/MATLAB Function7 ==
  data: t input; x_t output; T input; joy_position input; dx_t output; ddx_t output; N input
function [x_t, dx_t, ddx_t] = fcn(t, T, joy_position, N)
%#codegen
% Sliding-window waypoint planner:
% - Stores last N joystick positions as waypoints (uniformly spaced by T)
% - Generates a C2-continuous (pos/vel/acc) quintic segment between wp(:,1)->wp(:,2)
% - Boundary velocities/accelerations are NOT forced to zero; they are inferred
%   from the waypoint window (preview) and continuity is enforced by propagating
%   the end-state of the previous segment.

    % -------- Parameters (adjust maxN if you want bigger buffers) ----------
    maxN = 50;          % compile-time fixed buffer size
    Tmin = 1e-4;        % safety floor for T

    if T < Tmin
        T = Tmin;
    end

    % -------- Persistent state --------------------------------------------
    persistent wp              % 3 x maxN waypoint ring (we'll use first N columns)
    persistent seg_start_time
    persistent x_start dx_start ddx_start
    persistent x_target dx_target ddx_target
    persistent last_T Binv
    persistent initialized

    if isempty(initialized)
        initialized = true;

        % Clamp N to [1,maxN]
        if N < 1
            N = 1;
        elseif N > maxN
            N = maxN;
        end

        % Initialize waypoint buffer: replicate the initial joystick position
        wp = repmat(joy_position, 1, maxN);

        % Initialize segment start at current time
        seg_start_time = t;

        % Start state (you can set x_start=joy_position if you prefer)
        x_start   = wp(:,1);
        dx_start  = zeros(3,1);
        ddx_start = zeros(3,1);

        % Initial target is the "next" waypoint (same initially)
        x_target = wp(:,2);

        % Infer end derivatives from waypoint window (initially zeros)
        [dx_target, ddx_target] = inferEndDerivatives(wp, N, T);

        last_T = -1;
        Binv   = eye(3);
    end

    % Clamp N to [1,maxN] every call (robust to non-const input)
    if N < 1
        N = 1;
    elseif N > maxN
        N = maxN;
    end

    % -------- Cache inverse for this T ------------------------------------
    if isempty(last_T) || (T ~= last_T)
        T2 = T*T;  T3 = T2*T;
        T4 = T3*T; T5 = T4*T;

        b = [ T3,    T4,     T5;
             3*T2,  4*T3,   5*T4;
             6*T,  12*T2, 20*T3 ];

        Binv  = inv(b);
        last_T = T;
    end

    % -------- Segment time -------------------------------------------------
    t_segment = t - seg_start_time;

    % If time advanced past the segment end, advance segments robustly
    while t_segment >= T
        % End state of current segment at t = T (exact, for C2 continuity)
        [x_end, dx_end, ddx_end] = segment3D( ...
            x_start, dx_start, ddx_start, ...
            x_target, dx_target, ddx_target, ...
            T, T, Binv);

        % Promote end state -> new start state (guarantees C2 continuity)
        x_start   = x_end;
        dx_start  = dx_end;
        ddx_start = ddx_end;

        % Shift waypoint window left and append newest joystick sample
        % Use only the first N columns as the active window, but maintain maxN storage
        if N >= 2
            wp(:,1:N-1) = wp(:,2:N);
            wp(:,N)     = joy_position;
        else
            wp(:,1)     = joy_position;
        end

        % New target is next waypoint (wp(:,2)) if available, else current
        if N >= 2
            x_target = wp(:,2);
        else
            x_target = wp(:,1);
        end

        % Infer target end derivatives from waypoint window (no forcing to zero)
        [dx_target, ddx_target] = inferEndDerivatives(wp, N, T);

        % Advance segment start time
        seg_start_time = seg_start_time + T;
        t_segment = t - seg_start_time;
    end

    % Clamp within [0,T] to avoid extrapolation
    if t_segment < 0
        t_segment = 0;
    elseif t_segment > T
        t_segment = T;
    end

    % -------- Compute outputs in current segment ---------------------------
    [x_t, dx_t, ddx_t] = segment3D( ...
        x_start, dx_start, ddx_start, ...
        x_target, dx_target, ddx_target, ...
        T, t_segment, Binv);
end

% =========================================================================
function [dxT, ddxT] = inferEndDerivatives(wp, N, T)
% Estimate velocity/acceleration constraints at the END of the segment
% from the waypoint window (uniformly spaced by T).
%
% We plan from wp(:,1) -> wp(:,2). We infer desired derivatives at wp(:,2).
%
% - If N>=3: central-ish estimates using wp(:,1), wp(:,2), wp(:,3)
% - If N==2: first-difference velocity, zero accel
% - If N==1: zero vel/acc

    dxT  = zeros(3,1);
    ddxT = zeros(3,1);

    if N >= 3
        % Use wp1, wp2, wp3 to infer derivatives at wp2
        p1 = wp(:,1);
        p2 = wp(:,2);
        p3 = wp(:,3);

        % Velocity at p2 (symmetric difference around p2)
        dxT = (p3 - p1) / (2*T);

        % Acceleration at p2 (second difference)
        ddxT = (p3 - 2*p2 + p1) / (T*T);

    elseif N == 2
        p1 = wp(:,1);
        p2 = wp(:,2);

        dxT  = (p2 - p1) / T;
        ddxT = zeros(3,1);

    else
        dxT  = zeros(3,1);
        ddxT = zeros(3,1);
    end
end

% =========================================================================
function [x_t, dx_t, ddx_t] = segment3D(x0, dx0, ddx0, xT, dxT, ddxT, T, t, Binv)
    x_t   = zeros(3,1);
    dx_t  = zeros(3,1);
    ddx_t = zeros(3,1);

    for dim = 1:3
        [x_t(dim), dx_t(dim), ddx_t(dim)] = segment1D( ...
            x0(dim), dx0(dim), ddx0(dim), ...
            xT(dim), dxT(dim), ddxT(dim), ...
            T, t, Binv);
    end
end

% =========================================================================
function [x, dx, ddx] = segment1D(x0, dx0, ddx0, xT, dxT, ddxT, T, t, Binv)
% Quintic meeting (x,dx,ddx) at t=0 and t=T

    T2 = T*T;

    a1 = x0;
    a2 = dx0;
    a3 = ddx0/2;

    c1 = xT  - (a1 + a2*T + a3*T2);
    c2 = dxT - (a2 + 2*a3*T);
    c3 = ddxT - (2*a3);

    a456 = Binv * [c1; c2; c3];
    a4 = a456(1);
    a5 = a456(2);
    a6 = a456(3);

    t2 = t*t;  t3 = t2*t;  t4 = t3*t;  t5 = t4*t;

    x   = a1 + a2*t + a3*t2 + a4*t3 + a5*t4 + a6*t5;
    dx  = a2 + 2*a3*t + 3*a4*t2 + 4*a5*t3 + 5*a6*t4;
    ddx = 2*a3 + 6*a4*t + 12*a5*t2 + 20*a6*t3;
end
